simulink model "MPC"  (R2018a)
settings: Solver=FixedStepAuto  StartTime=0.0  StopTime=30  FixedStep=0.1  RelTol=1e-3
values from neighbouring files (symbols this model uses):
  a = 0.55    [Params.mat]
  Cf = 19000    [Params.mat]
  Cr = 33000    [Params.mat]
  deltau_max = 0.785398163397    [Params.mat]
  deltau_min = -0.785398163397    [Params.mat]
  dt = 0.1    [Params.mat]
  Iz = 2875    [Params.mat]
  lf = 1.2    [Params.mat]
  lr = 1.6    [Params.mat]
  m = 1575    [Params.mat]
  N = 10    [Params.mat]
  Nc = 3    [Params.mat]
  Np = 30    [Params.mat]
  u_max = 1.57079632679    [Params.mat]
  u_min = -1.57079632679    [Params.mat]
  y_max = 8    [Params.mat]
  y_min = -2    [Params.mat]
settings Model: Creator=yassine  LastModifiedBy=yassi
settings DataIOCC: ReturnWorkspaceOutputs=on
settings SFSimCC: SimUseLocalCustomCode=on
settings RTWCC: RTWUseLocalCustomCode=on

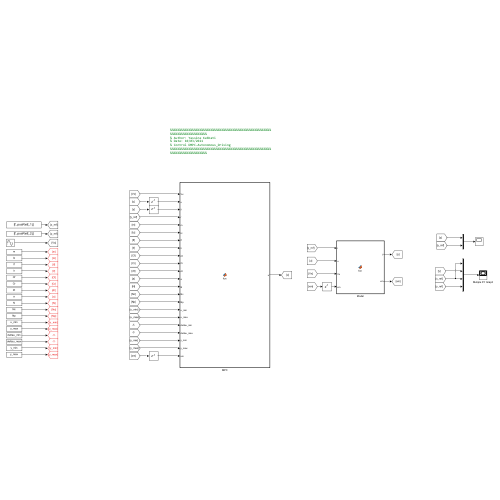
[thumbnail: Simulink's stored preview of the top-level diagram]
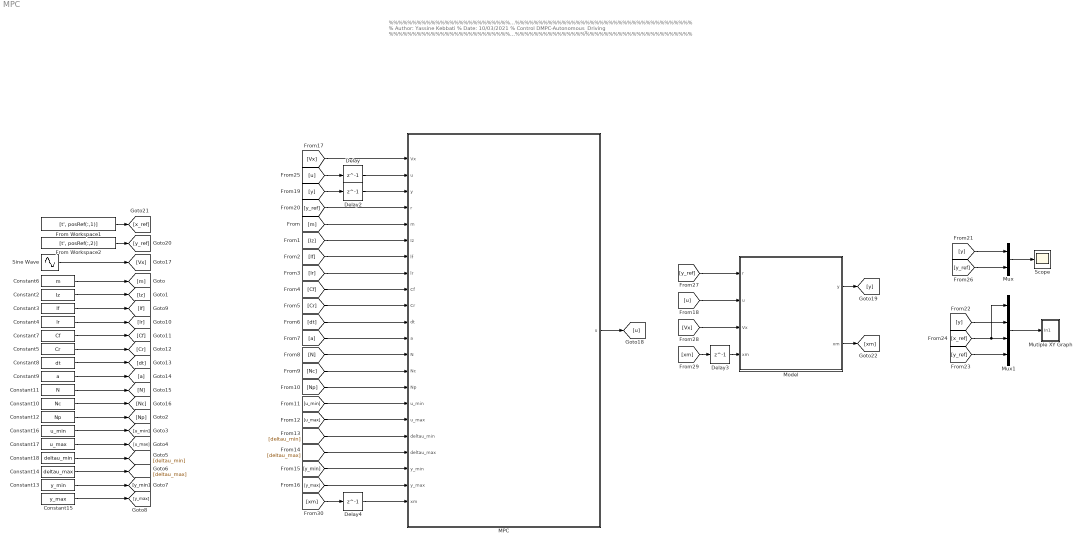
== system MPC ==
  note: %%%%%%%%%%%%%%%%%%%%%%%%%%%%%%%%%%%%%%%%%%%%%%%%%%%%%%%%%%%%%%%%%%%%%%%%%%%
      | % Author: Yassine Kebbati
      | % Date: 10/03/2021
      | % Control DMPC-Autonomous_Driving
      | %%%%%%%%%%%%%%%%%%%%%%%%%%%%%%%%%%%%%%%%%%%%%%%%%%%%%%%%%%%%%%%%%%%%%%%%%%%
  Constant10 : Constant  Value=Nc
  Constant11 : Constant  Value=N
  Constant12 : Constant  Value=Np
  Constant13 : Constant  Value=y_min
  Constant14 : Constant  Value=deltau_max
  Constant15 : Constant  Value=y_max
  Constant16 : Constant  Value=u_min
  Constant17 : Constant  Value=u_max
  Constant18 : Constant  Value=deltau_min
  Constant2 : Constant  Value=Iz
  Constant3 : Constant  Value=lf
  Constant4 : Constant  Value=lr
  Constant5 : Constant  Value=Cr
  Constant6 : Constant  Value=m
  Constant7 : Constant  Value=Cf
  Constant8 : Constant  Value=dt
  Constant9 : Constant  Value=a
  Delay{,2..4} (4 alike) : Delay  DelayLength=1
  From Workspace1 : FromWorkspace  VariableName=[t', posRef(:,1)]  SampleTime=0.1
  From Workspace2 : FromWorkspace  VariableName=[t', posRef(:,2)]  SampleTime=0.1
  MPC : MATLAB Function  TreatAsAtomicUnit=on
  Model : MATLAB Function  TreatAsAtomicUnit=on
  Mutiple XY Graph : Subsystem  mask(Mutiple XY Graph){number_of_trajectories=2, axis_limits=[0 320 -5 20], sample_time=0.1}
      mask prompts: number_of_trajectories "Number of Trajectories"; axis_limits "Axis Limits"; sample_time "Sample Time"
      mask Display: plot([.05 .95 .95 .05 .05],[.45 .45 .95 .95 .45], 0.5+cos(0:0.1:2*pi)*0.3,0.7+sin(0:0.1:2*pi)*0.2)
  Mux : Mux  Inputs=2
  Mux1 : Mux
  Scope : Scope
  Sine Wave : Sin  Amplitude=0  Bias=15  Frequency=0.8  SampleTime=0
  wires:
  [Vx] -> MPC/1(Vx)
  Delay/1 -> MPC/2("u ")
  [Cr] -> MPC/10(Cr)
  [lr] -> MPC/8(lr)
  [lf] -> MPC/7(lf)
  [Iz] -> MPC/6(Iz)
  [m] -> MPC/5(m)
  [Cf] -> MPC/9(Cf)
  [dt] -> MPC/11(dt)
  [a] -> MPC/12(a)
  [N] -> MPC/13(N)
  [Nc] -> MPC/14(Nc)
  [Np] -> MPC/15(Np)
  [u_max] -> MPC/17(u_max)
  [u_min] -> MPC/16(u_min)
  [deltau_min] -> MPC/18(deltau_min)
  [deltau_max] -> MPC/19(deltau_max)
  [y_min] -> MPC/20(y_min)
  [y_max] -> MPC/21(y_max)
  Delay2/1 -> MPC/3(y)
  Mux/1 -> Scope/1
  [y_ref] -> MPC/4(r)
  [x_ref] -> Mux1/1, Mux1/3
  Mux1/1 -> Mutiple XY Graph/1(In1)
  Constant15/1 -> [y_max]
  Constant6/1 -> [m]
  Constant2/1 -> [Iz]
  Constant3/1 -> [lf]
  Constant4/1 -> [lr]
  Constant7/1 -> [Cf]
  Constant5/1 -> [Cr]
  Constant8/1 -> [dt]
  Constant9/1 -> [a]
  Constant11/1 -> [N]
  Constant10/1 -> [Nc]
  Constant12/1 -> [Np]
  Constant16/1 -> [u_min]
  Constant17/1 -> [u_max]
  Constant18/1 -> [deltau_min]
  Constant14/1 -> [deltau_max]
  Constant13/1 -> [y_min]
  From Workspace2/1 -> [y_ref]
  Sine Wave/1 -> [Vx]
  Model/1(y) -> [y]
  [y] -> Mux/1
  [y] -> Mux1/2
  [y] -> Delay2/1
  [y_ref] -> Mux1/4
  From Workspace1/1 -> [x_ref]
  MPC/1(u) -> [u]
  [u] -> Model/2(u)
  [u] -> Delay/1
  [y_ref] -> Mux/2
  [y_ref] -> Model/1(r)
  [Vx] -> Model/3(Vx)
  Model/2(xm) -> [xm]
  [xm] -> Delay3/1
  Delay3/1 -> Model/4("xm ")
  [xm] -> Delay4/1
  Delay4/1 -> MPC/22(xm)

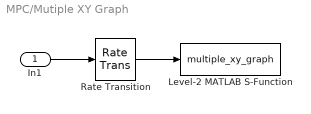
== system MPC/Mutiple XY Graph ==
  In1 : Inport
  Level-2 MATLAB S-Function : M-S-Function  FunctionName=multiple_xy_graph  Parameters=number_of_trajectories,axis_limits
  Rate Transition : RateTransition  OutPortSampleTime=sample_time
  wires:
  In1/1 -> Rate Transition/1
  Rate Transition/1 -> Level-2 MATLAB S-Function/1

== matlab function MPC/Model ==
  data: r input; u input; Vx input; y output size=[1,1]; xm input size=[4,1]; xm output size=[4,1]
%%%%%%%%%%%%%%%%%%%%%%%%%%%%%%%%%%%%%%%%%%%%%%%%%%%%%%%%%%%%%%%%%%%%%%%%%%%
% Author: Yassine Kebbati
% Date: 10/03/2021
% Control DMPC-Autonomous_Driving
%%%%%%%%%%%%%%%%%%%%%%%%%%%%%%%%%%%%%%%%%%%%%%%%%%%%%%%%%%%%%%%%%%%%%%%%%%%
function [y,xm] = fcn(r,u,Vx,xm)

coder.extrinsic('c2dm')

m = 1575;
Iz = 2875;
lf = 1.2;
lr = 1.6;
Cf = 19000;
Cr = 33000;

%persistent xm;
if isempty(xm)
  xm=[1.7628;0;0;0];
end

Ac = [-(2*Cf+2*Cr)/m/Vx, 0, -Vx-(2*Cf*lf-2*Cr*lr)/m/Vx, 0;
     0, 0, 1, 0;
     -(2*Cf*lf-2*Cr*lr)/Iz/Vx, 0, -(2*Cf*lf^2+2*Cr*lr^2)/Iz/Vx, 0;
     1, Vx, 0, 0];
Bc = [2*Cf/m 0 2*Cf*lf/Iz 0]';   
Cc = [0 0 0 1];
Dc = zeros(1,1);
Ad = zeros(4,4); Bd = zeros(4,1); Cd = zeros(1,4); Dd = zeros(1,1);
dt=0.1;
[Ad, Bd, Cd, Dd]=c2dm(Ac,Bc,Cc,Dc,dt,'zoh');


xm_old=xm;
xm=Ad*xm+Bd*u; % calculate xm(k+1)
y=Cd*xm; %calculate y(k+1)
o=0;

== matlab function MPC/MPC ==
  settings: updateMethod=DISCRETE
  data: u output; Vx input; u input; y input; r input; m input; Iz input; lf input; lr input; Cf input; Cr input; dt input; a input; N input; Nc input; Np input; u_min input; u_max input; deltau_min input; deltau_max input; y_min input; y_max input; xm input
%%%%%%%%%%%%%%%%%%%%%%%%%%%%%%%%%%%%%%%%%%%%%%%%%%%%%%%%%%%%%%%%%%%%%%%%%%%
% Author: Yassine Kebbati
% Date: 10/03/2021
% Control DMPC-Autonomous_Driving
%%%%%%%%%%%%%%%%%%%%%%%%%%%%%%%%%%%%%%%%%%%%%%%%%%%%%%%%%%%%%%%%%%%%%%%%%%%
function u = fcn(Vx, u,y,r,m,Iz,lf,lr,Cf,Cr,dt,a,N,Nc,Np,u_min,u_max,deltau_min,deltau_max,y_min,y_max,xm)



coder.extrinsic('c2dm')
%coder.extrinsic(function)

%load('new_trajectory.mat')


% Model identification

% m = 1575;
% Iz = 2875;
% lf = 1.2;
% lr = 1.6;
% Cf = 19000;
% Cr = 33000;



Ac = [-(2*Cf+2*Cr)/m/Vx, 0, -Vx-(2*Cf*lf-2*Cr*lr)/m/Vx, 0;
     0, 0, 1, 0;
     -(2*Cf*lf-2*Cr*lr)/Iz/Vx, 0, -(2*Cf*lf^2+2*Cr*lr^2)/Iz/Vx, 0;
     1, Vx, 0, 0];
Bc = [2*Cf/m 0 2*Cf*lf/Iz 0]';   
Cc = [0 0 0 1];
%C2 = [0 0 0 1; 0 1 0 0];
Dc = zeros(1,1);

%dt=0.1;
[Ad, Bd, Cd, Dd]=c2dm(Ac,Bc,Cc,Dc,dt,'zoh');
tic
% Make the augmented state-space model
n1 = 0;
m1 = 0;
n_in = 0;

[m1, n1] = size(Cd);
[n1, n_in] = size(Bd);
A = eye(n1+m1, n1+m1);
A(1:n1, 1:n1) = Ad;
A(n1+1:n1+m1,1:n1) = Cd*Ad;
B = zeros(n1+m1, n_in);
B(1:n1,:) = Bd;
B(n1+1:n1+m1,:) = Cd*Bd;
C = zeros(m1, n1+m1);
C(:, n1+1:n1+m1) = eye(m1, m1);
D = Dd;


% a=0.5;
% Nc=5;
% N=5; %you can increase N
% Np=25;

%obtain constraints data matrices

[M1,Lzerot]=Mdu(a,N,1,Nc);
M0=Mu(a,N,1,Nc);

%initial conditions for closed-loop simulation using constrained control
%specify the limits for ?u and u

%xm=zeros(n1,1);
% persistent xm;
% if isempty(xm)
%   xm=zeros(n1,1);
% end

persistent Xf
if isempty(Xf)
  Xf=[xm; y-r];
end

persistent xm_old
if isempty(xm_old)
  xm_old=zeros(4,1);
end
Xf=[xm-xm_old;y-r];
%end
xm_old=xm;

%specify constraints limits

% u_min=-pi/6;
% u_max=pi/6;
% deltau_min=-pi/12;
% deltau_max=pi/12;
% 
%  y_min=-2;
%  y_max=6;
y_bar_min=y_min-r;
y_bar_max=y_max-r;


%up=0.0;
up=u;

% C2 = [0 0 0 1; 0 1 0 0];
% Cc = [0 0 0 1];
% Generate matrices required for the predictive control cost function J

Q=C'*C;
R=0.0001;



%for kk=1:N_sim-1;
% Continuous-time model

% Ac = [-(2*Cf+2*Cr)/m, 0, -Vx-(2*Cf*lf-2*Cr*lr)/(m*Vx), 0;
%      0, 0, 1, 0;
%      -(2*Cf*lf-2*Cr*lr)/Iz/Vx, 0, -(2*Cf*lf^2+2*Cr*lr^2)/Iz/Vx, 0;
%      1, Vx, 0, 0];
% Bc = [2*Cf/m 0 2*Cf*lf/Iz 0]';   
% Cc = [0 0 0 1];
% C2 = [0 0 0 1; 0 1 0 0];
% Dc = zeros(1,1);

% Minimal realisation

% [num,den] = ss2tf(Ac,Bc,Cc,Dc);
% Gs = tf(num,den);
% 
% Gsmin=ss(Gs,'min');
% [Am,Bm,Cm,Dm]=ssdata(Gsmin);

% Discrete-time model

% dt=0.1;
% [Ad, Bd, Cd, Dd]=c2dm(Ac,Bc,Cc,Dc,dt,'zoh');

% Make the augmented state-space model

% [m1, n1] = size(Cd);
% [n1, n_in] = size(Bd);
% A = eye(n1+m1, n1+m1);
% A(1:n1, 1:n1) = Ad;
% A(n1+1:n1+m1,1:n1) = Cd*Ad;
% B = zeros(n1+m1, n_in);
% B(1:n1,:) = Bd;
% B(n1+1:n1+m1,:) = Cd*Bd;
% C = zeros(m1, n1+m1);
% C(:, n1+1:n1+m1) = eye(m1, m1);
% D = Dd;



[Phi,F]=mpcgain(Ad,Bd,Cd,N,Np);
[Omega,Psi]=dmpc(A,B,a,N,Np,Q,R);







%% constrains on U first
 M=[M0;-M0;M1;-M1;Phi(1:Nc,1)*Lzerot;-Phi(1:Nc,1)*Lzerot];


%closed-loop simulation performed recursively
%optimal control is also found recursively

%% constrains on u first
gamma=[(u_max-up)*ones(Nc,1);(-u_min+up)*ones(Nc,1);...
    deltau_max*ones(Nc,1);-deltau_min*ones(Nc,1);...
    y_bar_max-F(1:Nc,:)*Xf;-y_bar_min+F(1:Nc,:)*Xf];

eta=QPhild(Omega,Psi*Xf,M,gamma);

deltau=Lzerot*eta;
if (deltau>deltau_max) deltau=deltau_max;end
if (deltau<deltau_min) deltau=deltau_min;end
u=u+deltau;
if (u>u_max) deltau=u_max-up; u=u_max; end
if (u<u_min) deltau=u_min-up; u=u_min; end


%deltau1(1,kk)=deltau; %save data
%u1(1,kk)=u; %save data
%y1(:,kk)=y; %save data

%%%%
%plant simulation
%%%%%%


% xm=Ad*xm+Bd*u; % calculate xm(k+1)
% y=Cd*xm; %calculate y(k+1)
% y2=C2*xm;
% y3(1,kk)=y2(2,1);
% Xf=[xm-xm_old;y-r(1,kk)];
% y_bar_min=y_min-r(1,kk);
% y_bar_max=y_max-r(1,kk);

timeElapsed = toc
